simulink subsystem "PowerUnit_AMK"  (R2021b)
settings: Solver=VariableStepAuto  StartTime=0.0  StopTime=10.0  RelTol=1e-3
libraries: simulink x9
settings Model: Creator=tsuyoshi  LastModifiedBy=tsuyoshi

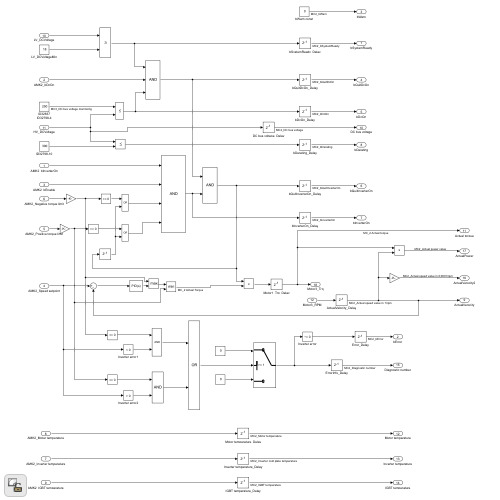
[thumbnail: Simulink's stored preview of the top-level diagram]
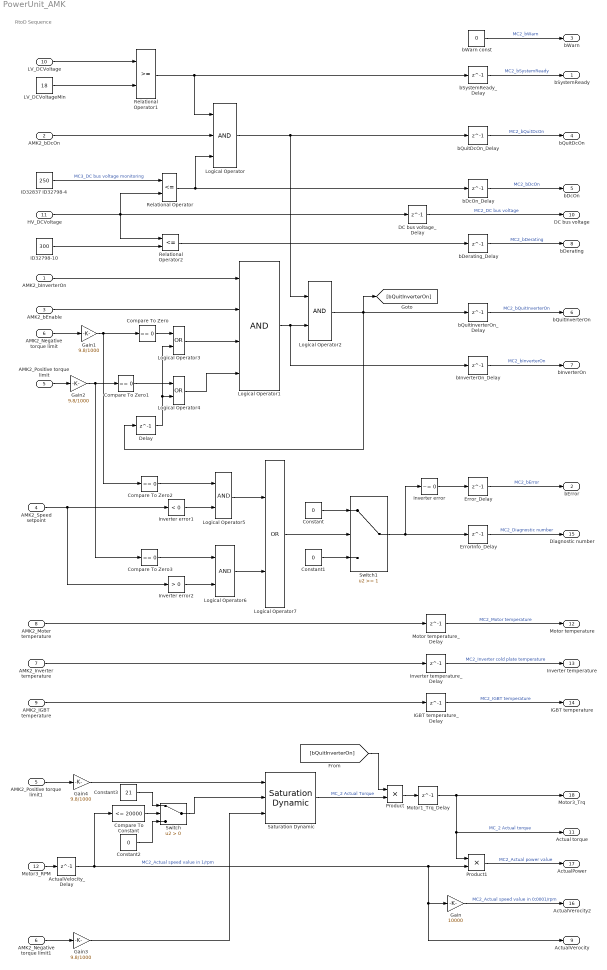
== system PowerUnit_AMK ==
  note: RtoD Sequence
  AMK2_bInverterOn : Inport
  AMK2_bDcOn : Inport  Port=2
  AMK2_bEnable : Inport  Port=3
  AMK2_Speed setpoint : Inport  Port=4
  AMK2_Positive torque limit : Inport  Port=5
  AMK2_Negative torque limit : Inport  Port=6
  AMK2_Inverter temperature : Inport  Port=7
  AMK2_Moter temperature : Inport  Port=8
  AMK2_IGBT temperature : Inport  Port=9
  LV_DCVoltage : Inport  Port=10
  HV_DCVoltage : Inport  Port=11
  Motor3_RPM : Inport  Port=12
  AMK2_Negative torque limit1 : InportShadow  Port=6
  AMK2_Positive torque limit1 : InportShadow  Port=5
  ActualVelocity_Delay : Delay  DelayLength=1  InitialCondition=0
  Compare To Constant : simulink/Logic and Bit Operations/Compare To Constant  relop=<=  const=20000  OutDataTypeStr=boolean
  Compare To Zero{,1..3} (4 alike) : simulink/Logic and Bit Operations/Compare To Zero  relop===  OutDataTypeStr=boolean
  Constant : Constant  Value=0
  Constant1 : Constant  Value=0
  Constant2 : Constant  Value=0
  Constant3 : Constant  Value=21
  DC bus voltage_Delay : Delay  DelayLength=1  InitialCondition=0
  Delay : Delay  DelayLength=1  InitialCondition=0
  ErrorInfo_Delay : Delay  DelayLength=1  InitialCondition=0
  Error_Delay : Delay  DelayLength=1  InitialCondition=0
  Gain : Gain  Gain=10000
  Gain{1..4} (4 alike) : Gain  Gain=9.8/1000
  ID32798-10 : Constant  Value=300
  ID32837 ID32798-4 : Constant  Value=250
  IGBT temperature_Delay : Delay  DelayLength=1  InitialCondition=0
  Inverter error : simulink/Logic and Bit Operations/Compare To Zero  relop=~=  OutDataTypeStr=boolean
  Inverter error1 : simulink/Logic and Bit Operations/Compare To Zero  relop=<  OutDataTypeStr=boolean
  Inverter error2 : simulink/Logic and Bit Operations/Compare To Zero  relop=>  OutDataTypeStr=boolean
  Inverter temperature_Delay : Delay  DelayLength=1  InitialCondition=0
  LV_DCVoltageMin : Constant  Value=18
  Logical Operator : Logic  Inputs=3  AllPortsSameDT=off  OutDataTypeStr=boolean
  Logical Operator1 : Logic  Inputs=4  AllPortsSameDT=off  OutDataTypeStr=boolean
  Logical Operator2 : Logic  AllPortsSameDT=off  OutDataTypeStr=boolean
  Logical Operator3 : Logic  Operator=OR  AllPortsSameDT=off  OutDataTypeStr=boolean
  Logical Operator4 : Logic  Operator=OR  AllPortsSameDT=off  OutDataTypeStr=boolean
  Logical Operator5 : Logic  AllPortsSameDT=off  OutDataTypeStr=boolean
  Logical Operator6 : Logic  AllPortsSameDT=off  OutDataTypeStr=boolean
  Logical Operator7 : Logic  Operator=OR  AllPortsSameDT=off  OutDataTypeStr=boolean
  Motor temperature_Delay : Delay  DelayLength=1  InitialCondition=0
  Motor1_Trq_Delay : Delay  DelayLength=1  InitialCondition=0
  Product : Product
  Product1 : Product
  Relational Operator : RelationalOperator  Operator=<=  OutDataTypeStr=boolean  RndMeth=Simplest
  Relational Operator1 : RelationalOperator  OutDataTypeStr=boolean  RndMeth=Simplest
  Relational Operator2 : RelationalOperator  Operator=<=  OutDataTypeStr=boolean  RndMeth=Simplest
  Saturation Dynamic : simulink/Discontinuities/Saturation Dynamic  OutMin=[]  OutMax=[]  OutDataTypeStr=Inherit: Same as second input  OutDataType=fixdt(1, 16)  OutScaling=2^-10  DoSatur=off
  Switch : Switch  Criteria=u2 > Threshold
  Switch1 : Switch  Threshold=1
  bDcOn_Delay : Delay  DelayLength=1  InitialCondition=0
  bDerating_Delay : Delay  DelayLength=1  InitialCondition=0
  bInverterOn_Delay : Delay  DelayLength=1  InitialCondition=0
  bQuitDcOn_Delay : Delay  DelayLength=1  InitialCondition=0
  bQuitInverterOn_Delay : Delay  DelayLength=1  InitialCondition=0
  bSystemReady_Delay : Delay  DelayLength=1  InitialCondition=0
  bWarn const : Constant  Value=0
  bSystemReady : Outport  VectorParamsAs1DForOutWhenUnconnected=off
  bError : Outport  Port=2  VectorParamsAs1DForOutWhenUnconnected=off
  bWarn : Outport  Port=3  VectorParamsAs1DForOutWhenUnconnected=off
  bQuitDcOn : Outport  Port=4  VectorParamsAs1DForOutWhenUnconnected=off
  bDcOn : Outport  Port=5  VectorParamsAs1DForOutWhenUnconnected=off
  bQuitInverterOn : Outport  Port=6  VectorParamsAs1DForOutWhenUnconnected=off
  bInverterOn : Outport  Port=7  VectorParamsAs1DForOutWhenUnconnected=off
  bDerating : Outport  Port=8  VectorParamsAs1DForOutWhenUnconnected=off
  ActualVerocity : Outport  Port=9  VectorParamsAs1DForOutWhenUnconnected=off
  DC bus voltage : Outport  Port=10  VectorParamsAs1DForOutWhenUnconnected=off
  Actual torque : Outport  Port=11  VectorParamsAs1DForOutWhenUnconnected=off
  Motor temperature : Outport  Port=12  VectorParamsAs1DForOutWhenUnconnected=off
  Inverter temperature : Outport  Port=13  VectorParamsAs1DForOutWhenUnconnected=off
  IGBT temperature : Outport  Port=14  VectorParamsAs1DForOutWhenUnconnected=off
  Diagnostic number : Outport  Port=15  VectorParamsAs1DForOutWhenUnconnected=off
  ActualVerocity2 : Outport  Port=16  VectorParamsAs1DForOutWhenUnconnected=off
  ActualPower : Outport  Port=17  VectorParamsAs1DForOutWhenUnconnected=off
  Motor3_Trq : Outport  Port=18  VectorParamsAs1DForOutWhenUnconnected=off
  wires:
  Logical Operator6/1 -> Logical Operator7/2
  Logical Operator3/1 -> Logical Operator1/3
  AMK2_bInverterOn/1 -> Logical Operator1/1
  AMK2_IGBT temperature/1 -> IGBT temperature_Delay/1
  LV_DCVoltageMin/1 -> Relational Operator1/2
  AMK2_bDcOn/1 -> Logical Operator/2
  Relational Operator1/1 -> Logical Operator/1, bSystemReady_Delay/1
  Logical Operator/1 -> Logical Operator2/1, bQuitDcOn_Delay/1
  LV_DCVoltage/1 -> Relational Operator1/1
  Relational Operator/1 -> Logical Operator/3, bDcOn_Delay/1
  Relational Operator2/1 -> bDerating_Delay/1
  ID32837 ID32798-4/1 -> Relational Operator/1  "MC3_DC bus voltage monitoring"
  AMK2_Negative torque limit/1 -> Gain1/1
  HV_DCVoltage/1 -> Relational Operator/2, DC bus voltage_Delay/1, Relational Operator2/1
  AMK2_Moter temperature/1 -> Motor temperature_Delay/1
  ID32798-10/1 -> Relational Operator2/2
  Logical Operator1/1 -> Logical Operator2/2, bInverterOn_Delay/1
  Compare To Zero/1 -> Logical Operator3/1
  Logical Operator2/1 -> bQuitInverterOn_Delay/1, [bQuitInverterOn], Delay/1
  AMK2_Inverter temperature/1 -> Inverter temperature_Delay/1
  AMK2_bEnable/1 -> Logical Operator1/2
  Compare To Zero1/1 -> Logical Operator4/1
  AMK2_Positive torque limit/1 -> Gain2/1
  AMK2_Speed setpoint/1 -> Inverter error1/1, Inverter error2/1
  Constant1/1 -> Switch1/3
  Logical Operator7/1 -> Switch1/2
  Logical Operator4/1 -> Logical Operator1/4
  Compare To Zero3/1 -> Logical Operator6/1
  Constant/1 -> Switch1/1
  Logical Operator5/1 -> Logical Operator7/1
  Compare To Zero2/1 -> Logical Operator5/1
  Delay/1 -> Logical Operator4/2, Logical Operator3/2
  Switch1/1 -> Inverter error/1, ErrorInfo_Delay/1
  bSystemReady_Delay/1 -> bSystemReady/1  "MC2_bSystemReady"
  bQuitDcOn_Delay/1 -> bQuitDcOn/1  "MC2_bQuitDcOn"
  bDcOn_Delay/1 -> bDcOn/1  "MC2_bDcOn"
  bDerating_Delay/1 -> bDerating/1  "MC2_bDerating"
  bQuitInverterOn_Delay/1 -> bQuitInverterOn/1  "MC2_bQuitInverterOn"
  bInverterOn_Delay/1 -> bInverterOn/1  "MC2_bInverterOn"
  ActualVelocity_Delay/1 -> Compare To Constant/1, Product1/2, Gain/1, ActualVerocity/1  "MC2_Actual speed value in 1/rpm"
  ErrorInfo_Delay/1 -> Diagnostic number/1  "MC2_Diagnostic number"
  Motor temperature_Delay/1 -> Motor temperature/1  "MC2_Motor temperature"
  Inverter temperature_Delay/1 -> Inverter temperature/1  "MC2_Inverter cold plate temperature"
  IGBT temperature_Delay/1 -> IGBT temperature/1  "MC2_IGBT temperature"
  Inverter error/1 -> Error_Delay/1
  Error_Delay/1 -> bError/1  "MC2_bError"
  DC bus voltage_Delay/1 -> DC bus voltage/1  "MC2_DC bus voltage"
  bWarn const/1 -> bWarn/1  "MC2_bWarn"
  Gain/1 -> ActualVerocity2/1  "MC2_Actual speed value in 0;0001/rpm"
  Product1/1 -> ActualPower/1  "MC2_Actual power value"
  Inverter error1/1 -> Logical Operator5/2
  Inverter error2/1 -> Logical Operator6/2
  Product/1 -> Motor1_Trq_Delay/1
  Motor3_RPM/1 -> ActualVelocity_Delay/1
  Motor1_Trq_Delay/1 -> Motor3_Trq/1, Actual torque/1, Product1/1  "MC_2 Actual torque"
  Gain1/1 -> Compare To Zero2/1, Compare To Zero/1
  Gain2/1 -> Compare To Zero1/1, Compare To Zero3/1
  Switch/1 -> Saturation Dynamic/2
  Saturation Dynamic/1 -> Product/2  "MC_2 Actual Torque"
  AMK2_Negative torque limit1/1 -> Gain3/1
  Gain3/1 -> Saturation Dynamic/3
  AMK2_Positive torque limit1/1 -> Gain4/1
  Gain4/1 -> Saturation Dynamic/1
  [bQuitInverterOn] -> Product/1
  Compare To Constant/1 -> Switch/2
  Constant2/1 -> Switch/3
  Constant3/1 -> Switch/1
